simulink model "Modelo_final"  (R2023b)
settings: Solver=VariableStepAuto  StartTime=0.0  StopTime=60  RelTol=1e-3
libraries: SignalEditorBlockLib x3
settings Model: Creator=sebaschitiva  LastModifiedBy=sebaschitiva

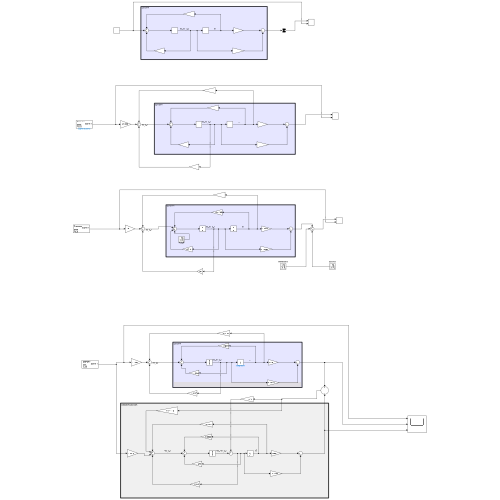
[thumbnail: Simulink's stored preview of the top-level diagram]
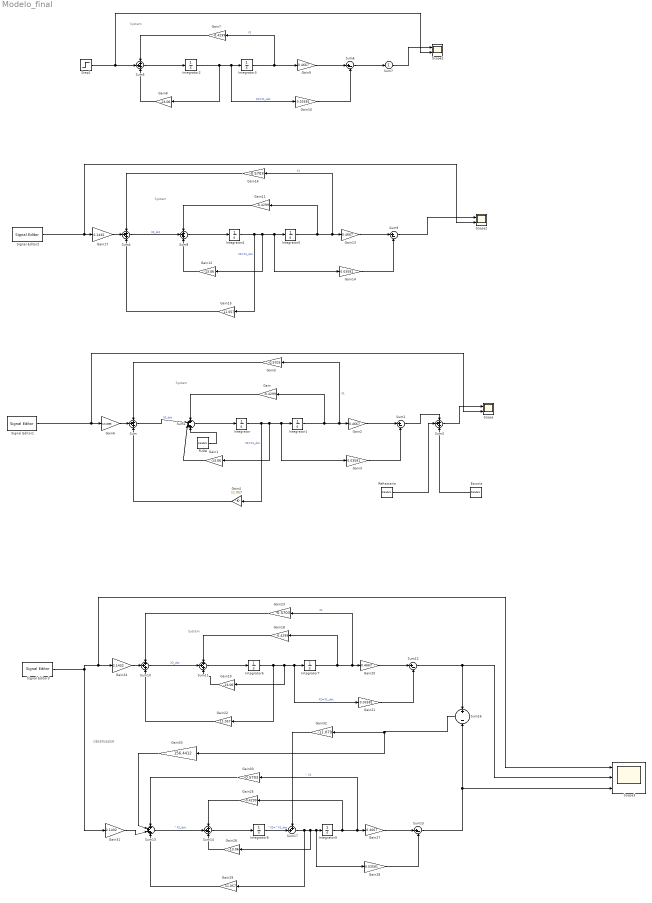
== system Modelo_final ==
  note: OBSERVADOR
  note: System
  note: System
  note: System
  note: System
  Escoria : RandomNumber  Mean=-1.5  Variance=2.25  Seed=123435  SampleTime=0.1
  FUGA : RandomNumber  Seed=12345  SampleTime=0.1
  Gain{,7,11,18,25} (5 alike) : Gain  Gain=-0.4299
  Gain{1,8,12,19,26} (5 alike) : Gain  Gain=-13.06
  Gain{3,10,14,21,28} (5 alike) : Gain  Gain=0.03581
  Gain{2,9,13,20,27} (5 alike) : Gain  Gain=0.4667
  Gain{4,15,22,29} (4 alike) : Gain  Gain=11.057
  Gain{5,16,23,30} (4 alike) : Gain  Gain=-0.5703
  Gain17 : Gain  Gain=2.1432
  Gain24 : Gain  Gain=2.1432
  Gain31 : Gain  Gain=2.1432
  Gain32 : Gain  Gain=-11.079
  Gain33 : Gain  Gain=156.4412
  Gain6 : Gain  Gain=1/0.4666
  Integrator{,1..9} (10 alike) : Integrator
  Refractario : RandomNumber  Variance=4.0  Seed=67890  SampleTime=0.1
  Scope : Scope  NumInputPorts=2
  Scope1 : Scope  NumInputPorts=2
  Scope2 : Scope  NumInputPorts=2
  Scope3 : Scope  NumInputPorts=3
  Signal Editor1 : SignalEditorBlockLib/Signal Editor  FileName=/Users/sebaschitiva/Desktop/Prueba/sim1.mat  ActiveScenario=Scenario  ActiveSignal=Signal 1  IsBus=off  OutputBusObjectStr=Bus: BusObject  SampleTime=0  Interpolate=off  ZeroCross=off  OutputAfterFinalValue=Setting to zero  Unit=inherit  PreserveSignalName=on  ApplySigPropsToAllScenarios=on  ApplySigPropsToAllSignals=off
  Signal Editor2 : SignalEditorBlockLib/Signal Editor  FileName=/Users/sebaschitiva/Desktop/Prueba/sim1.mat  ActiveScenario=Scenario  ActiveSignal=Signal 1  IsBus=off  OutputBusObjectStr=Bus: BusObject  SampleTime=0  Interpolate=off  ZeroCross=off  OutputAfterFinalValue=Setting to zero  Unit=inherit  PreserveSignalName=on  ApplySigPropsToAllScenarios=on  ApplySigPropsToAllSignals=off
  Signal Editor3 : SignalEditorBlockLib/Signal Editor  FileName=/Users/sebaschitiva/Desktop/Prueba/sim1.mat  ActiveScenario=Scenario  ActiveSignal=Signal 1  IsBus=off  OutputBusObjectStr=Bus: BusObject  SampleTime=0  Interpolate=off  ZeroCross=off  OutputAfterFinalValue=Setting to zero  Unit=inherit  PreserveSignalName=on  ApplySigPropsToAllScenarios=on  ApplySigPropsToAllSignals=off
  Step1 : Step  Time=0  SampleTime=0
  Sum{,3..5,8,10..11,14} (8 alike) : Sum  Inputs=+++
  Sum1 : Sum  Inputs=++++
  Sum{2,6,9,12,15} (5 alike) : Sum  Inputs=|+-
  Sum13 : Sum  Inputs=++++
  Sum16 : Sum  Inputs=+-
  Sum17 : Sum  Inputs=++|
  Sum7 : Sum  Inputs=+
  wires:
  Signal Editor1/1 -> Gain6/1, Scope/2
  Gain/1 -> Sum1/1
  Gain1/1 -> Sum1/3
  Sum1/1 -> Integrator/1
  Integrator/1 -> Gain4/1, Gain1/1, Gain3/1, Integrator1/1  "X2=X1_dot"
  Integrator1/1 -> Gain/1, Gain5/1, Gain2/1  "X1"
  Gain2/1 -> Sum2/1
  Gain3/1 -> Sum2/2
  Gain4/1 -> Sum/3
  Gain5/1 -> Sum/1
  Sum/1 -> Sum1/2  "X2_dot"
  Gain6/1 -> Sum/2
  Sum3/1 -> Scope/1
  Sum2/1 -> Sum3/1
  Refractario/1 -> Sum3/2
  Gain10/1 -> Sum6/2
  Sum7/1 -> Scope1/1
  Integrator3/1 -> Gain7/1, Gain9/1  "X1"
  Gain7/1 -> Sum5/1
  Gain8/1 -> Sum5/3
  Integrator2/1 -> Gain8/1, Gain10/1, Integrator3/1  "X2=X1_dot"
  Gain9/1 -> Sum6/1
  Sum5/1 -> Integrator2/1
  Step1/1 -> Scope1/2, Sum5/2
  Sum6/1 -> Sum7/1
  FUGA/1 -> Sum1/4
  Escoria/1 -> Sum3/3
  Gain14/1 -> Sum9/2
  Gain16/1 -> Sum4/1
  Integrator5/1 -> Gain11/1, Gain16/1, Gain13/1  "X1"
  Gain11/1 -> Sum8/1
  Gain12/1 -> Sum8/3
  Integrator4/1 -> Gain15/1, Gain12/1, Gain14/1, Integrator5/1  "X2=X1_dot"
  Gain13/1 -> Sum9/1
  Gain15/1 -> Sum4/3
  Sum8/1 -> Integrator4/1
  Sum4/1 -> Sum8/2  "X2_dot"
  Gain17/1 -> Sum4/2
  Signal Editor2/1 -> Scope2/2, Gain17/1
  Sum9/1 -> Scope2/1
  Gain22/1 -> Sum10/3
  Integrator7/1 -> Gain18/1, Gain23/1, Gain20/1  "X1"
  Gain18/1 -> Sum11/1
  Gain20/1 -> Sum12/1
  Gain23/1 -> Sum10/1
  Gain19/1 -> Sum11/3
  Gain24/1 -> Sum10/2
  Integrator6/1 -> Gain22/1, Gain19/1, Gain21/1, Integrator7/1  "X2=X1_dot"
  Sum10/1 -> Sum11/2  "X2_dot"
  Gain21/1 -> Sum12/2
  Sum11/1 -> Integrator6/1
  Gain26/1 -> Sum14/3
  Sum13/1 -> Sum14/2  "^X2_dot"
  Integrator8/1 -> Sum17/2  "^X2=^X1_dot"
  Gain25/1 -> Sum14/1
  Gain30/1 -> Sum13/1
  Sum14/1 -> Integrator8/1
  Signal Editor3/1 -> Scope3/1, Gain24/1, Gain31/1
  Sum15/1 -> Scope3/3, Sum16/2
  Gain28/1 -> Sum15/2
  Gain27/1 -> Sum15/1
  Integrator9/1 -> Gain25/1, Gain30/1, Gain27/1  "^ X1"
  Sum16/1 -> Gain33/1, Gain32/1
  Gain32/1 -> Sum17/1
  Sum17/1 -> Gain29/1, Gain28/1, Integrator9/1, Gain26/1
  Gain29/1 -> Sum13/4
  Gain31/1 -> Sum13/3
  Gain33/1 -> Sum13/2
  Sum12/1 -> Sum16/1, Scope3/2
